simulink model "MuscleModel_ThelenRigidInverse"  (R2024b)
settings: Solver=VariableStepAuto  StartTime=0.0  StopTime=10.0  RelTol=1e-3
undefined symbols (not defined in the file or in its folder): alpha0, LM0, LTs
settings Model: Creator=jakub  LastModifiedBy=jakub

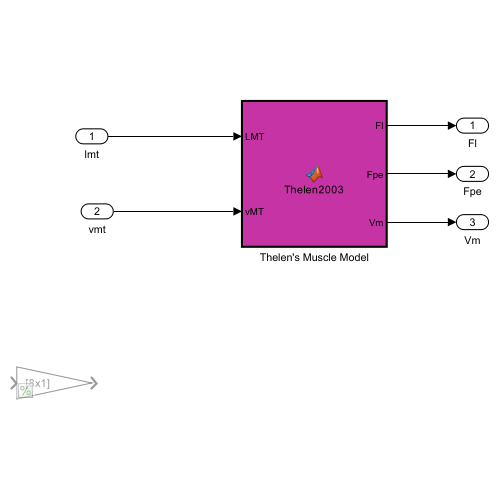
[thumbnail: Simulink's stored preview of the top-level diagram]
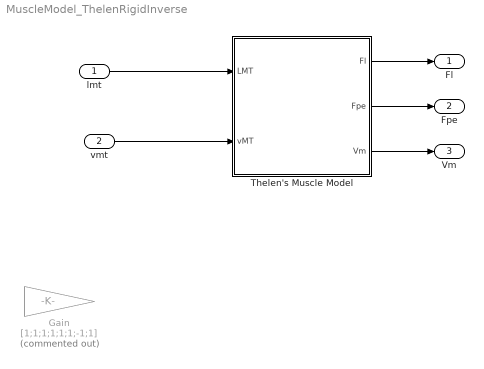
== system MuscleModel_ThelenRigidInverse ==
  lmt : Inport  OutDataTypeStr=double  Unit=m  PortDimensions=[8 1]  SampleTime=0
  vmt : Inport  Port=2  OutDataTypeStr=double  Unit=m/s  PortDimensions=[8 1]  SampleTime=0
  Gain : Gain  Commented=on  Gain=[1;1;1;1;1;1;-1;1]
  Thelen's Muscle Model : MATLAB Function  TreatAsAtomicUnit=on
  Fl : Outport  OutDataTypeStr=double  PortDimensions=[8 1]  SampleTime=0
  Fpe : Outport  Port=2  OutDataTypeStr=double  PortDimensions=[8 1]  SampleTime=0
  Vm : Outport  Port=3  OutDataTypeStr=double  Unit=m/s  PortDimensions=[8 1]  SampleTime=0
  wires:
  lmt/1 -> Thelen's Muscle Model/1(LMT)
  Thelen's Muscle Model/1(Fl) -> Fl/1
  Thelen's Muscle Model/2(Fpe) -> Fpe/1
  Thelen's Muscle Model/3(Vm) -> Vm/1
  vmt/1 -> Thelen's Muscle Model/2(vMT)

== matlab function MuscleModel_ThelenRigidInverse/Thelen's Muscle Model ==
  data: LMT input double size=[8 1]; vMT input double size=[8 1]; Fl output double size=[8 1]; LM0 parameter double size=[8 1]; LTs parameter double size=[8 1]; Fpe output double size=[8 1]; Vm output double size=[8 1]; alpha0 parameter
function [Fl, Fpe, Vm]  = Thelen2003(LMT, vMT, LM0, LTs, alpha0)

    % Muscle constants
        epsM0 = 0.6;            % passive muscle strain due to maximum isometric force
        kPE = 4;                % an exponential shape factor for the passive force-length relationship
        gamma = 0.5;            % a shape factor for the Gaussian active force-length relationship

    Fl = zeros(numel(LM0),1);
    Fpe = zeros(numel(LM0),1);
    Vm = zeros(numel(LM0),1);
    
    for k = 1:numel(LM0)
        Lmt = LMT(k);
        Lt = LTs(k);
        Lm0 = LM0(k);
        vmt = vMT(k);
        alpha = alpha0(k);


    %% Muscle length and velocity
        Lm = (Lmt - Lt)/cos(alpha);
        vm = vmt*cos(alpha);

        lm = Lm/Lm0;

    %% Force of the (contractile element) - ACTIVE FORCE
        fl = exp(-(lm-1)^2/gamma);
    
    %% Force of the muscle parallel element - PASSIVE FORCE
        fpe = (exp(kPE*(lm - 1)/epsM0) - 1) / (exp(kPE) - 1);
        if fpe < 0
            fpe = 0;
        end

    %% OUTPUT
        Fpe(k) = fpe;
        Fl(k) = fl;
        Vm(k) = vm;
    end
end
